simulink model "env_environment_model_hrn"  (R2015a)
settings: Solver=ode3  StartTime=0.0  StopTime=sim_end_time  FixedStep=.01  RelTol=1e-3
libraries: env_environment_model_lib x1
settings Model: CovSFcnEnable=off  Creator=jfusco1  LastModifiedBy=rhnakamu
settings DebuggingCC: SolverPrmCheckMsg=warning

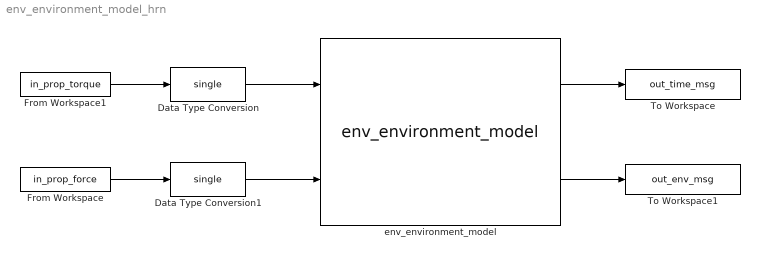
== system env_environment_model_hrn ==
  Data Type Conversion : DataTypeConversion  OutDataTypeStr=single
  Data Type Conversion1 : DataTypeConversion  OutDataTypeStr=single
  From Workspace : FromWorkspace  VariableName=in_prop_force  SampleTime=0  Interpolate=off  OutputAfterFinalValue=Holding final value
  From Workspace1 : FromWorkspace  VariableName=in_prop_torque  SampleTime=0  Interpolate=off  OutputAfterFinalValue=Holding final value
  To Workspace : ToWorkspace  VariableName=out_time_msg  SaveFormat=Timeseries  SampleTime=-1
  To Workspace1 : ToWorkspace  VariableName=out_env_msg  SaveFormat=Timeseries  SampleTime=-1
  env_environment_model : env_environment_model_lib/env_environment_model  VariantControl=(default)
  wires:
  From Workspace/1 -> Data Type Conversion1/1
  From Workspace1/1 -> Data Type Conversion/1
  env_environment_model/1 -> To Workspace/1
  env_environment_model/2 -> To Workspace1/1
  Data Type Conversion/1 -> env_environment_model/1
  Data Type Conversion1/1 -> env_environment_model/2
